simulink model "ModeloHibrido"  (R2023b)
settings: Solver=VariableStepAuto  StartTime=0.0  StopTime=10.0  RelTol=1e-3
settings Model: Creator=USUARIO  LastModifiedBy=USUARIO

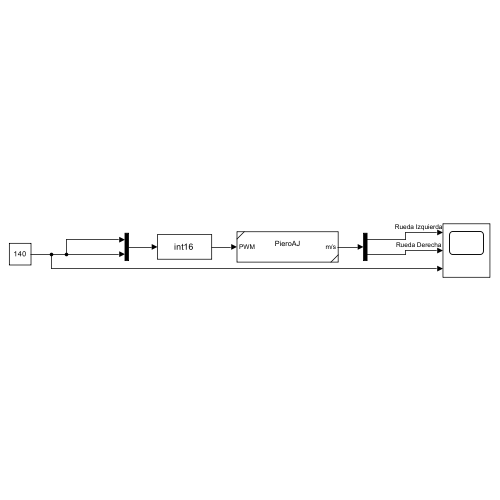
[thumbnail: Simulink's stored preview of the top-level diagram]
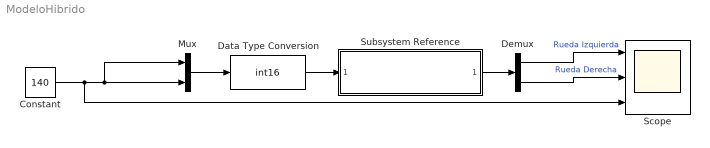
== system ModeloHibrido ==
  Constant : Constant  Value=140
  Data Type Conversion : DataTypeConversion  OutDataTypeStr=int16  SaturateOnIntegerOverflow=off  RndMeth=Floor
  Demux : Demux  Outputs=2
  Mux : Mux  Inputs=2
  Scope : Scope  NumInputPorts=3
  Subsystem Reference : Subsystem  ReferencedSubsystem=PieroAJ
  wires:
  Data Type Conversion/1 -> Subsystem Reference/1
  Constant/1 -> Scope/3, Mux/1, Mux/2
  Mux/1 -> Data Type Conversion/1
  Subsystem Reference/1 -> Demux/1
  Demux/1 -> Scope/1  "Rueda Izquierda"
  Demux/2 -> Scope/2  "Rueda Derecha"
